simulink model "WMR_Trajectory_Tracking"  (R2016b)
settings: Solver=VariableStepAuto  StartTime=0.0  StopTime=200  RelTol=1e-3
undefined symbols (not defined in the file): kd1, kd2, kp1, kp2, R, Tc, thetai, vi, xi, yi
libraries: simulink x2
settings Model: Creator=Bryce  LastModifiedBy=Bryce

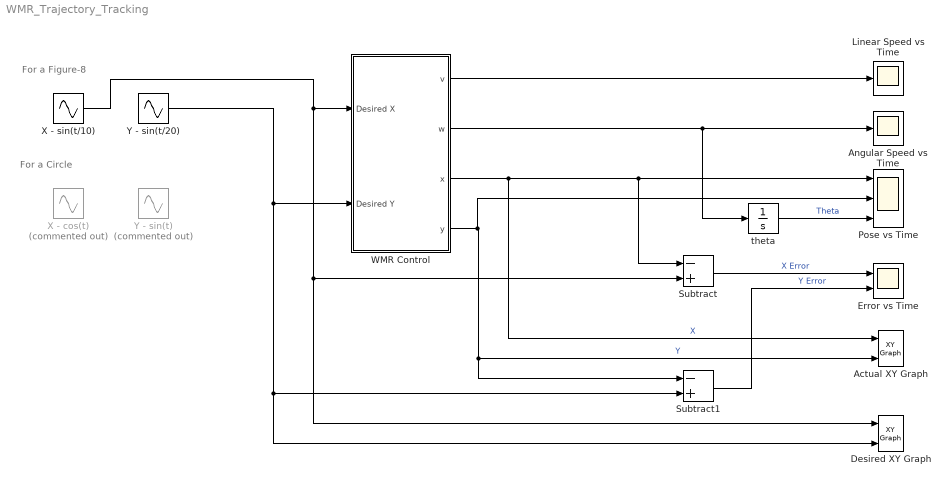
== system WMR_Trajectory_Tracking ==
  note: For a Circle
  note: For a Figure-8
  Actual XY Graph : simulink/Sinks/XY Graph  xmin=-R  xmax=R  ymin=-R  ymax=R  st=-1
  Angular Speed vs Time : Scope
  Desired XY Graph : simulink/Sinks/XY Graph  xmin=-R  xmax=R  ymin=-R  ymax=R  st=-1
  Error vs Time : Scope  NumInputPorts=2
  Linear Speed vs Time : Scope
  Pose vs Time : Scope  NumInputPorts=3
  Subtract : Sum  Inputs=-+
  Subtract1 : Sum  Inputs=-+
  WMR Control : Subsystem
  X - cos(t) : Sin  Commented=on  Phase=pi/2  SampleTime=0
  X - sin(t/10) : Sin  Frequency=1/10  SampleTime=0
  Y - sin(t) : Sin  Commented=on  SampleTime=0
  Y - sin(t/20) : Sin  Frequency=1/20  SampleTime=0
  theta : Integrator
  wires:
  WMR Control/1(v) -> Linear Speed vs Time/1
  WMR Control/2(w) -> theta/1, Angular Speed vs Time/1
  WMR Control/3(x) -> Actual XY Graph/1, Subtract/1, Pose vs Time/1  "X"
  WMR Control/4(y) -> Pose vs Time/2, Subtract1/1, Actual XY Graph/2  "Y"
  Subtract/1 -> Error vs Time/1  "X Error"
  Subtract1/1 -> Error vs Time/2  "Y Error"
  theta/1 -> Pose vs Time/3  "Theta"
  Y - sin(t/20)/1 -> Subtract1/2, Desired XY Graph/2, WMR Control/2(Desired Y)
  X - sin(t/10)/1 -> Subtract/2, Desired XY Graph/1, WMR Control/1(Desired X)

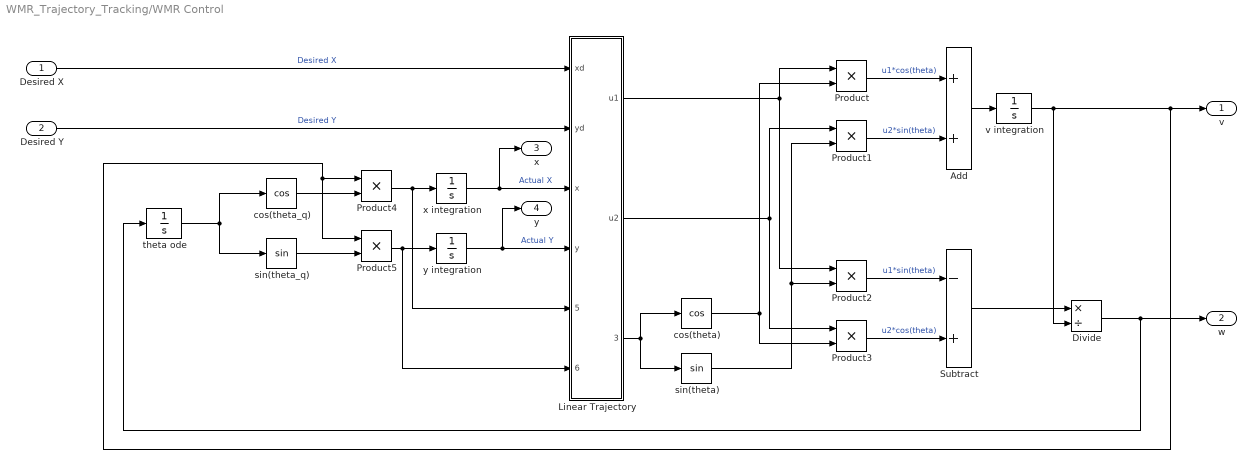
== system WMR_Trajectory_Tracking/WMR Control ==
  Desired X : Inport
  Desired Y : Inport  Port=2
  Add : Sum
  Divide : Product  Inputs=*/
  Linear Trajectory : Subsystem
  Product{,1..5} (6 alike) : Product
  Subtract : Sum  Inputs=-+
  cos(theta) : Trigonometry  Operator=cos
  cos(theta_q) : Trigonometry  Operator=cos
  sin(theta) : Trigonometry
  sin(theta_q) : Trigonometry
  theta ode : Integrator  InitialCondition=thetai
  v integration : Integrator  InitialCondition=vi
  x integration : Integrator  InitialCondition=xi
  y integration : Integrator  InitialCondition=yi
  v : Outport
  w : Outport  Port=2
  x : Outport  Port=3
  y : Outport  Port=4
  wires:
  x integration/1 -> Linear Trajectory/3(x), x/1  "Actual X"
  y integration/1 -> Linear Trajectory/4(y), y/1  "Actual Y"
  Linear Trajectory/1(u1) -> Product/1, Product2/1
  cos(theta)/1 -> Product/2, Product3/2
  Linear Trajectory/2(u2) -> Product1/1, Product3/1
  sin(theta)/1 -> Product2/2, Product1/2
  Product/1 -> Add/1  "u1*cos(theta)"
  Product1/1 -> Add/2  "u2*sin(theta)"
  Product3/1 -> Subtract/2  "u2*cos(theta)"
  Product2/1 -> Subtract/1  "u1*sin(theta)"
  Subtract/1 -> Divide/1
  Divide/1 -> w/1, theta ode/1
  Product5/1 -> y integration/1, Linear Trajectory/6(y_dot)
  Linear Trajectory/3(theta) -> sin(theta)/1, cos(theta)/1
  Product4/1 -> x integration/1, Linear Trajectory/5(x_dot)
  sin(theta_q)/1 -> Product5/2
  cos(theta_q)/1 -> Product4/2
  Add/1 -> v integration/1
  v integration/1 -> Product5/1, Product4/1, v/1, Divide/2
  Desired X/1 -> Linear Trajectory/1(xd)  "Desired X"
  Desired Y/1 -> Linear Trajectory/2(yd)  "Desired Y"
  theta ode/1 -> sin(theta_q)/1, cos(theta_q)/1

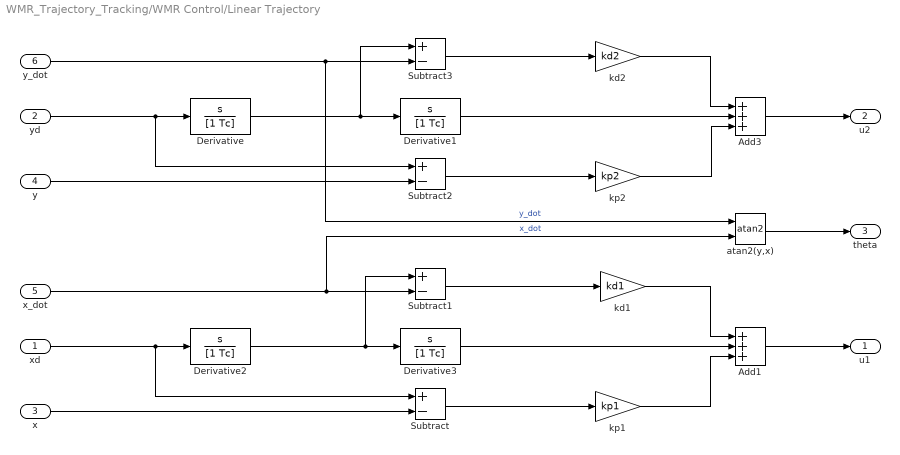
== system WMR_Trajectory_Tracking/WMR Control/Linear Trajectory ==
  xd : Inport
  yd : Inport  Port=2
  x : Inport  Port=3
  y : Inport  Port=4
  x_dot : Inport  Port=5
  y_dot : Inport  Port=6
  Add1 : Sum  Inputs=+++
  Add3 : Sum  Inputs=+++
  Derivative{,1..3} (4 alike) : TransferFcn  Numerator=[1 0]  Denominator=[1 Tc]
  Subtract{,1..3} (4 alike) : Sum  Inputs=+-
  atan2(y,x) : Trigonometry  Operator=atan2
  kd1 : Gain  Gain=kd1
  kd2 : Gain  Gain=kd2
  kp1 : Gain  Gain=kp1
  kp2 : Gain  Gain=kp2
  u1 : Outport
  u2 : Outport  Port=2
  theta : Outport  Port=3
  wires:
  xd/1 -> Derivative2/1, Subtract/1
  Subtract1/1 -> kd1/1
  Add3/1 -> u2/1
  x/1 -> Subtract/2
  Subtract/1 -> kp1/1
  x_dot/1 -> atan2(y,x)/2, Subtract1/2  "x_dot"
  kd1/1 -> Add1/1
  kp1/1 -> Add1/3
  Subtract3/1 -> kd2/1
  y/1 -> Subtract2/2
  Subtract2/1 -> kp2/1
  kd2/1 -> Add3/1
  kp2/1 -> Add3/3
  Add1/1 -> u1/1
  atan2(y,x)/1 -> theta/1
  y_dot/1 -> atan2(y,x)/1, Subtract3/2  "y_dot"
  yd/1 -> Derivative/1, Subtract2/1
  Derivative/1 -> Derivative1/1, Subtract3/1
  Derivative1/1 -> Add3/2
  Derivative3/1 -> Add1/2
  Derivative2/1 -> Derivative3/1, Subtract1/1
